simulink model "complex_UIO_2"  (R2019b)
settings: Solver=FixedStepAuto  StartTime=0.0  StopTime=60  FixedStep=0.1  RelTol=1e-3
values from neighbouring files (symbols this model uses):
  Ac = [real(A) -imag(A);imag(A) real(A)]    [DAC_UIO_Comp.m]    (also in LinearND_QUANTUM_2020_11_14_2.m = [realA -imagA;imagA realA]; UIO_alternative_2021_01_26.m; UIO_alternative_PAPER_2021_02_17.m = Abar(2:3,2:3); UIO_alternative_PAPER_2021_03_01.m = Abar(2:3,2:3))
  Amc = [real(Am) -imag(Am);imag(Am) real(Am)]    [DAC_UIO_Comp.m]    (also in UIO_alternative_2021_01_26.m)
  Bc = [real(B) -imag(B);imag(B) real(B)]    [DAC_UIO_Comp.m]    (also in UIO_alternative_2021_01_26.m; UIO_alternative_PAPER_2021_02_17.m = Bbar(2:3,:); UIO_alternative_PAPER_2021_03_01.m = Bbar(2:3,:))
  C = double(subs(C_sym,{ep},{0.1}))    [DAC_UIO_Comp.m]    (also in UIO_adaptive_example.m = [1 0 0 0 0;0 0 0 1 0; 0 0 0 0 1]; UIO_adaptive_example_2.m = [1 0 0 0;0 1 0 0]; UIO_adaptive_example_EEG_Balas_2ch.m = [1, epsilon]; UIO_adaptive_example_alternative_EEG_ch6.m = ss_c.C)
  g1 = 4+2j    [DAC_UIO_Comp.m]    (also in UIO_adaptive_example_EEG_Balas_2ch.m = 4; UIO_alternative_2021_01_26.m = 2+1j; UIO_alternative_PAPER_2021_02_17.m = 2; UIO_alternative_PAPER_2021_03_01.m = 2)
  g2 = 0    [DAC_UIO_Comp.m]    (also in UIO_adaptive_example_EEG_Balas_2ch.m = -0.3; UIO_alternative_2021_01_26.m; UIO_alternative_PAPER_2021_02_17.m = 1; UIO_alternative_PAPER_2021_03_01.m)
  g3 = 0    [DAC_UIO_Comp.m]    (also in UIO_adaptive_example_EEG_Balas_2ch.m = 0.1; UIO_alternative_2021_01_26.m; UIO_alternative_PAPER_2021_02_17.m = -3; UIO_alternative_PAPER_2021_03_01.m)
  gamma_e = 1    [DAC_UIO_Comp.m]    (also in UIO_adaptive_example_EEG_Balas_2ch.m; UIO_adaptive_example_alternative_EEG_ch6.m = .0001*ones(length(Am),1); UIO_alternative_2021_01_26.m = 0.001; UIO_alternative_PAPER_2021_02_17.m = 0.0001)
  gamma_u = 1    [DAC_UIO_Comp.m]    (also in UIO_adaptive_example_EEG_Balas_2ch.m = 2)
settings Model: Creator=Tris  LastModifiedBy=Tris

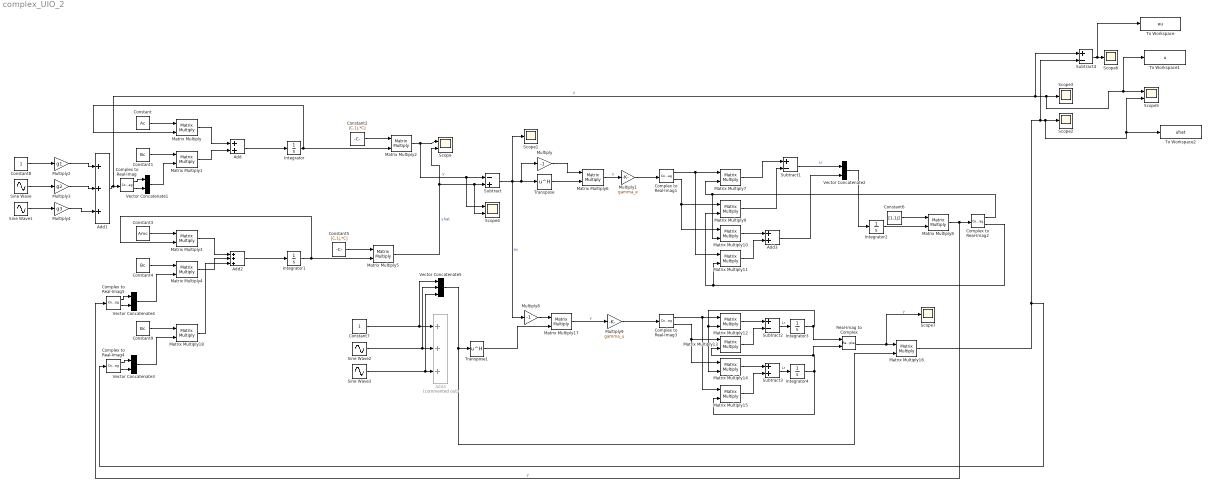
== system complex_UIO_2 ==
  Add : Sum
  Add1 : Sum  Inputs=+++
  Add2 : Sum  Inputs=+++
  Add3 : Sum
  Add4 : Sum  Commented=on  Inputs=+++
  Complex to Real-Imag{,1..5} (6 alike) : ComplexToRealImag
  Constant : Constant  Value=Ac
  Constant1 : Constant  Value=Bc  VectorParams1D=off
  Constant2 : Constant  Value=[C,1j.*C]  VectorParams1D=off
  Constant3 : Constant  Value=Amc
  Constant4 : Constant  Value=Bc  VectorParams1D=off
  Constant5 : Constant  Value=[C,1j.*C]  VectorParams1D=off
  Constant6 : Constant  Value=[1,1j]  VectorParams1D=off
  Constant7 : Constant  VectorParams1D=off
  Constant8 : Constant  VectorParams1D=off
  Constant9 : Constant  Value=Bc  VectorParams1D=off
  Integrator : Integrator
  Integrator1 : Integrator
  Integrator2 : Integrator  InitialCondition=[1;0.5]
  Integrator3 : Integrator  InitialCondition=[-1,-1,-1]
  Integrator4 : Integrator  InitialCondition=[-1,-1,-1]
  Matrix Multiply{,1..18} (19 alike) : Product  Multiplication=Matrix(*)
  Multiply : Gain  Gain=-1
  Multiply1 : Gain  Gain=gamma_e
  Multiply2 : Gain  Gain=g1
  Multiply3 : Gain  Gain=g2
  Multiply4 : Gain  Gain=g3
  Multiply8 : Gain  Gain=-1
  Multiply9 : Gain  Gain=gamma_u
  Real-Imag to Complex : RealImagToComplex
  Scope : Scope  NumInputPorts=2
  Scope{1..3,6..7} (5 alike) : Scope
  Scope4 : Scope  NumInputPorts=2
  Scope5 : Scope  NumInputPorts=2
  Sine Wave : Sin  SampleTime=0  VectorParams1D=off
  Sine Wave1 : Sin  Phase=pi/2  SampleTime=0  VectorParams1D=off
  Sine Wave2 : Sin  SampleTime=0  VectorParams1D=off
  Sine Wave3 : Sin  Phase=pi/2  SampleTime=0  VectorParams1D=off
  Subtract : Sum  Inputs=-+
  Subtract1 : Sum  Inputs=+-
  Subtract2 : Sum  Inputs=+-
  Subtract3 : Sum
  Subtract4 : Sum  Inputs=+-
  To Workspace : ToWorkspace  VariableName=eu  SaveFormat=Timeseries  SampleTime=-1
  To Workspace1 : ToWorkspace  VariableName=u  SaveFormat=Timeseries  SampleTime=-1
  To Workspace2 : ToWorkspace  VariableName=uhat  SaveFormat=Timeseries  SampleTime=-1
  Transpose : Math  Operator=hermitian  SignedPower=off  SaturateOnIntegerOverflow=on
  Transpose1 : Math  Operator=hermitian  SignedPower=off  SaturateOnIntegerOverflow=on
  Vector Concatenate{1..4} (4 alike) : Concatenate  Mode=Multidimensional array
  Vector Concatenate5 : Concatenate  NumInputs=3  Mode=Multidimensional array
  wires:
  Constant/1 -> Matrix Multiply/1
  Integrator/1 -> Matrix Multiply2/2, Matrix Multiply/2
  Add/1 -> Integrator/1
  Matrix Multiply/1 -> Add/1
  Matrix Multiply1/1 -> Add/2
  Constant1/1 -> Matrix Multiply1/1
  Multiply4/1 -> Add1/3
  Multiply3/1 -> Add1/2
  Multiply2/1 -> Add1/1
  Sine Wave1/1 -> Multiply4/1
  Constant8/1 -> Multiply2/1
  Sine Wave/1 -> Multiply3/1
  Constant2/1 -> Matrix Multiply2/1
  Add1/1 -> Subtract4/1, To Workspace1/1, Scope5/1, Scope3/1, Complex to Real-Imag/1  "u"
  Complex to Real-Imag/1 -> Vector Concatenate1/1
  Complex to Real-Imag/2 -> Vector Concatenate1/2
  Vector Concatenate1/1 -> Matrix Multiply1/2
  Matrix Multiply2/1 -> Scope4/1, Subtract/1, Scope/1  "y"
  Constant3/1 -> Matrix Multiply3/1
  Matrix Multiply3/1 -> Add2/1
  Matrix Multiply4/1 -> Add2/2
  Constant4/1 -> Matrix Multiply4/1
  Add2/1 -> Integrator1/1
  Integrator1/1 -> Matrix Multiply5/2, Matrix Multiply3/2
  Constant5/1 -> Matrix Multiply5/1
  Matrix Multiply5/1 -> Scope/2, Scope4/2, Subtract/2  "yhat"
  Subtract/1 -> Multiply8/1, Multiply/1, Transpose/1, Scope1/1  "ey"
  Transpose/1 -> Matrix Multiply6/2
  Multiply/1 -> Matrix Multiply6/1
  Matrix Multiply6/1 -> Multiply1/1  "y"
  Multiply1/1 -> Complex to Real-Imag1/1
  Complex to Real-Imag1/1 -> Matrix Multiply11/1, Matrix Multiply7/1
  Complex to Real-Imag1/2 -> Matrix Multiply10/1, Matrix Multiply9/1
  Vector Concatenate2/1 -> Integrator2/1
  Integrator2/1 -> Matrix Multiply8/2
  Constant6/1 -> Matrix Multiply8/1
  Matrix Multiply8/1 -> Complex to Real-Imag5/1, Complex to Real-Imag2/1  "y"
  Complex to Real-Imag2/1 -> Matrix Multiply7/2, Matrix Multiply10/2
  Matrix Multiply7/1 -> Subtract1/1
  Matrix Multiply9/1 -> Subtract1/2
  Complex to Real-Imag2/2 -> Matrix Multiply11/2, Matrix Multiply9/2
  Subtract1/1 -> Vector Concatenate2/1  "Lr"
  Matrix Multiply10/1 -> Add3/1
  Add3/1 -> Vector Concatenate2/2
  Matrix Multiply11/1 -> Add3/2
  Sine Wave2/1 -> Vector Concatenate5/2, Add4/2
  Sine Wave3/1 -> Vector Concatenate5/3, Add4/3
  Constant7/1 -> Vector Concatenate5/1, Add4/1
  Multiply9/1 -> Complex to Real-Imag3/1
  Transpose1/1 -> Matrix Multiply17/2
  Multiply8/1 -> Matrix Multiply17/1
  Matrix Multiply17/1 -> Multiply9/1  "y"
  Complex to Real-Imag5/2 -> Vector Concatenate4/2
  Vector Concatenate4/1 -> Matrix Multiply4/2
  Complex to Real-Imag5/1 -> Vector Concatenate4/1
  Vector Concatenate5/1 -> Transpose1/1, Matrix Multiply16/2
  Complex to Real-Imag3/1 -> Matrix Multiply15/1, Matrix Multiply12/1
  Matrix Multiply12/1 -> Subtract2/1
  Subtract2/1 -> Integrator3/1  "Lr"
  Integrator3/1 -> Real-Imag to Complex/1, Matrix Multiply14/2, Matrix Multiply12/2
  Matrix Multiply13/1 -> Subtract2/2
  Matrix Multiply14/1 -> Subtract3/1
  Matrix Multiply15/1 -> Subtract3/2
  Subtract3/1 -> Integrator4/1  "Lr"
  Integrator4/1 -> Matrix Multiply15/2, Real-Imag to Complex/2, Matrix Multiply13/2
  Real-Imag to Complex/1 -> Scope7/1, Matrix Multiply16/1  "y"
  Complex to Real-Imag3/2 -> Matrix Multiply14/1, Matrix Multiply13/1
  Subtract4/1 -> To Workspace/1, Scope6/1
  Constant9/1 -> Matrix Multiply18/1
  Vector Concatenate3/1 -> Matrix Multiply18/2
  Complex to Real-Imag4/1 -> Vector Concatenate3/1
  Complex to Real-Imag4/2 -> Vector Concatenate3/2
  Matrix Multiply18/1 -> Add2/3
  Matrix Multiply16/1 -> Subtract4/2, To Workspace2/1, Scope5/2, Scope2/1, Complex to Real-Imag4/1
